simulink model "Model_Main_V2"  (R2019b)
settings: Solver=FixedStepAuto  StartTime=0.0  StopTime=inf  RelTol=1e-3  EnableMultiTasking=on
PreLoadFcn:
  | sampleTime = 0.01;
  | 
  | % Vehicle Parameters
  | R = 0.058;
  | L = 0.1;
  | vehicle = DifferentialDrive(R,L);
  | k = -858.9174;
  | b = 70.9944;
  | %model parameters
  | MODEL_TYPE = 0;
  | MODEL_TYPE_ROAD = 0;
InitFcn:
  | sampleTime = 0.01;
  | 
  | % Vehicle Parameters
  | R = 0.058;
  | L = 0.1;
  | vehicle = DifferentialDrive(R,L);
  | k = -858.9174;
  | b = 70.9944;
undefined symbols (not defined in the file or in its folder): DiscIntNeverNeededParam, InitAngle, InitX
libraries: legoev3lib x5, mobileRoboticsLib x4, aerolibconvert2 x3, simulink x2
settings Model: ExtModeTrigDuration=2  Creator=nikit  LastModifiedBy=nikit
settings SolverCC: PositivePriorityOrder=on
settings OptimizationCC: EnhancedBackFolding=on  PassReuseOutputArgsAs=Individual arguments  ZeroExternalMemoryAtStartup=off  ZeroInternalMemoryAtStartup=off  MaxStackSize=64  OptimizeBlockOrder=speed  DifferentSizesBufferReuse=on  EfficientTunableParamExpr=on
settings DebuggingCC: ParameterTunabilityLossMsg=error
settings HardwareCC: ProdBitPerPointer=32  ProdBitPerSizeT=32  ProdBitPerPtrDiffT=32  ProdLargestAtomicInteger=Long  ProdWordSize=32  ProdHWDeviceType=ARM Compatible->ARM 9
settings SFSimCC: MATLABDynamicMemAlloc=off
settings RTWCC: SystemTargetFile=ert.tlc  HardwareBoard=LEGO MINDSTORMS EV3  TLCOptions="-aInlineSetEventsForThisBaseRateFcn=TLC_FALSE -aSuppressMultiTaskScheduler=TLC_FALSE  -aRateBasedStepFcn=0"  TemplateMakefile=ert_default_tmf  GenerateReport=on  Toolchain=Sourcery G++ Lite v2009q3  IncludeHyperlinkInReport=on  LaunchReport=on  GenerateTraceInfo=on  GenerateTraceReport=on  GenerateTraceReportSl=on  GenerateTraceReportSf=on  GenerateTraceReportEml=on
settings CodeAppCC: ForceParamTrailComments=on  IgnoreCustomStorageClasses=off  OperatorAnnotations=on  SimulinkDataObjDesc=on  SFDataObjDesc=on  InsertBlockDesc=on
settings ERTTargetCC: SupportContinuousTime=on  SupportVariableSizeSignals=on

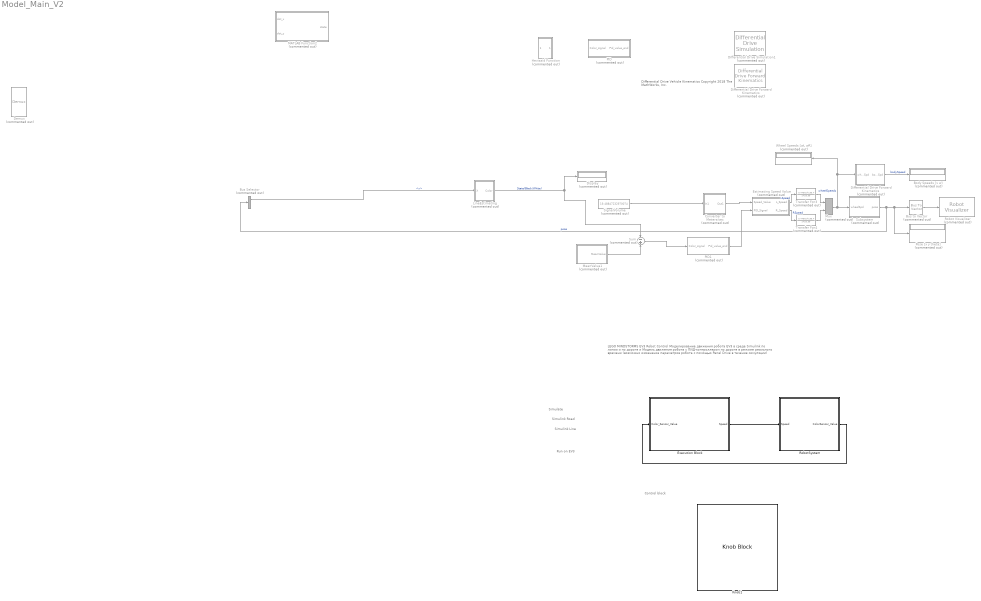
== system Model_Main_V2 ==
  note: LEGO MINDSTORMS EV3 Robot Control
      | Моделирование движения робота EV3 в среде Simulink по линии и по дороге
      | и
      | Модель движения робота с ПИД-контроллером по дороге в режиме реального времени
      | (возможно изменение параметров робота с помощью Panel Drive в течение симуляции)
  note: Simulate
  note: Run on EV3
  note: Simulink Road
  note: Control block
  note: Differential Drive Vehicle Kinematics
      |
      | Copyright 2018 The MathWorks, Inc.
  note: Simulink Line
  Body Speeds [v w] : Display  Commented=on
  Bus Selector : BusSelector  Commented=on  OutputSignals=x,y,ang
  Bus to Vector : BusToVector  Commented=on
  Converter to Meters/sec : Subsystem  Commented=on
  Demux : Demux  Commented=on  Outputs=3
  Differential Drive Forward Kinematics : mobileRoboticsLib/Kinematic Models/Differential Drive/Differential Drive Forward Kinematics  Commented=on  wheelRadius=R  wheelBase=L
      settings: SourceProductName=Mobile Robotics Simulation Library
  Differential Drive Forward Kinematics : Subsystem  Commented=on  AncestorBlock=mobileRoboticsLib/Kinematic Models/Differential Drive/Differential Drive Forward Kinematics  mask(Differential Drive Forward Kinematics){wheelRadius=R, wheelBase=L}
      mask prompts: wheelRadius "Wheel Radius [m]"; wheelBase "Wheelbase [m]"
      mask help:
      | Calculates the forward kinematics for a differential drive vehicle.
      |
      | Input: [wL; wR], the left and right wheel speeds (rad/s)
      |
      | Output: [v; w], the linear (m/s) and angular (rad/s) velocities of the vehicle
      mask Help: web('matlab:edit mrsDocDifferentialDrive')
  Differential Drive Simulation1 : mobileRoboticsLib/Kinematic Models/Differential Drive/Differential Drive Simulation  Commented=on  wheelRadius=R  wheelBase=L  initX=0  initY=18  initAngle=0  Ts=0.01
      link override Differential Drive  Forward Kinematics: wheelRadius=R  wheelBase=L
      link override Generic Robot Simulation: initX=initX  initY=initY  initAngle=initAngle
      settings: SourceProductName=Mobile Robotics Simulation Library
  Display : Display  Commented=on
  Estimating Speed Value : Subsystem  Commented=on
  Execution Block : Subsystem
      mask Display: image('ev3_computer.jpg'); % Use "Edit Image" on toolstrip to change.
  "Hevisaid Function " : Subsystem  Commented=on
  Knob1 : KnobBlock
  LineEstimating : Subsystem  Commented=on
  MATLAB Function2 : MATLAB Function  Commented=on  TreatAsAtomicUnit=on
  MeanValue1 : Subsystem  Commented=on  mask{BlackCode=3, WhiteCode=32}
      mask prompts: BlackCode "BlackColorCode"; WhiteCode "WhiteColorCode"
  Mux : Mux  Commented=on  Inputs=2
  PID : Subsystem  Commented=on
  PID1 : Subsystem  Commented=on
  Pose [x y theta] : Display  Commented=on
  Robot Visualizer : mobileRoboticsLib/Environments/Robot Visualizer  Priority=99  Commented=on  robotRadius=0.15  mapName=map  showTrajectory=on  hasWaypoints=off  hasLidar=off  sensorOffset=[ 0 0 ]  scanAngles=scanAngles  hasObjDetector=off  objDetectorOffset=[ 0, 0 ]  objDetectorAngle=0  objDetectorFOV=pi/4  objDetectorMaxRange=5  objectColors=[ 1, 0, 0; 0, 1, 0; 0, 0, 1 ]  objectMarkers=s
      settings: SourceProductName=Mobile Robotics Simulation Library
  RobotSystem : Subsystem  Variant=on  VariantControl=Variant1
      mask Display:
      | if evalin('base','MODEL_TYPE == 1')
      |     image('EV3_Robot.jpg')
      | else
      |     image('ev3_simulink_sign.jpg')
      | end
  SignalVolume : Constant  Commented=on  Value=19.48847232970074
  Subsystem : Subsystem  Commented=on  mask{R=0.058, L=0.155, InitialX=0.6455, InitialY=0.02, InitialAngle=pi/2, SampleTime=0.01}
      mask prompts: R "WheelR"; L "BodyL"; InitialAngle "InitialAng"; SampleTime "Sample Time"
  Sum : Sum  Commented=on  Inputs=-+
  Transfer Fcn3 : TransferFcn  Commented=on  Numerator=[0.4456 195.4]  Denominator=[1 20.39]
  Transfer Fcn4 : TransferFcn  Commented=on  Numerator=[0.4456 195.4]  Denominator=[1 20.39]
  Wheel Speeds [wL wR] : Display  Commented=on
  wires:
  LineEstimating/1(Color) -> Sum/1, Display/1  "State(Black/White)"
  MeanValue1/1(MeanValue) -> Sum/2
  Estimating Speed Value/1(L_Speed) -> Transfer Fcn3/1  "LSpeed"
  Estimating Speed Value/2(R_Speed) -> Transfer Fcn4/1  "RSpeed"
  Differential Drive Forward Kinematics/1(bodySpd) -> Body Speeds [v w]/1  "bodySpeed"
  Mux/1 -> Subsystem/1(wheelSpd), Differential Drive Forward Kinematics/1(wheelSpd), Wheel Speeds [wL wR]/1  "wheelSpeeds"
  Subsystem/1(pose) -> Pose [x y theta]/1, Bus to Vector/1, Bus Selector/1  "pose"
  Converter to Meters/sec/1(Out1) -> Estimating Speed Value/1(Speed_Value)
  Bus to Vector/1 -> Robot Visualizer/1
  PID1/1(Pid_value_end) -> Estimating Speed Value/2(PID_Signal)
  Bus Selector/1 -> LineEstimating/1(X)  "<x>"
  Sum/1 -> PID1/1(Color_signal)
  SignalVolume/1 -> Converter to Meters/sec/1(In1)
  Transfer Fcn3/1 -> Mux/1
  Transfer Fcn4/1 -> Mux/2
  RobotSystem/1(ColorSensor_Value) -> Execution Block/1(Color_Sensor_Value)
  Execution Block/1(Speed) -> RobotSystem/1(Speed)

== system Model_Main_V2/Converter to Meters//sec ==
  In1 : Inport
  Angle Conversion : aerolibconvert2/Angle Conversion  IU=deg  OU=rad
  Radius : Gain  Gain=R
  Out1 : Outport
  wires:
  Radius/1 -> Out1/1
  Angle Conversion/1 -> Radius/1
  In1/1 -> Angle Conversion/1

== system Model_Main_V2/Differential Drive Forward Kinematics ==
  wheelSpd : Inport
  Demux : Demux  Outputs=2
  ForwardKinematics : Subsystem
  Mux : Mux  Inputs=2
  bodySpd : Outport  VectorParamsAs1DForOutWhenUnconnected=off
  wires:
  Demux/2 -> ForwardKinematics/2(wR)  "wR"
  Demux/1 -> ForwardKinematics/1(wL)  "wL"
  wheelSpd/1 -> Demux/1
  Mux/1 -> bodySpd/1
  ForwardKinematics/2(w) -> Mux/2  "w"
  ForwardKinematics/1(v) -> Mux/1  "v"

== system Model_Main_V2/Estimating Speed Value ==
  note: Estimating Speed Value for each engine taking into account PID_value
  Speed_Value : Inport
  PID_Signal : Inport  Port=2
  Sum1 : Sum  Inputs=+-|
  Sum2 : Sum  Inputs=++|
  L_Speed : Outport
  R_Speed : Outport  Port=2
  wires:
  Speed_Value/1 -> Sum2/1, Sum1/1
  PID_Signal/1 -> Sum2/2, Sum1/2
  Sum2/1 -> R_Speed/1
  Sum1/1 -> L_Speed/1

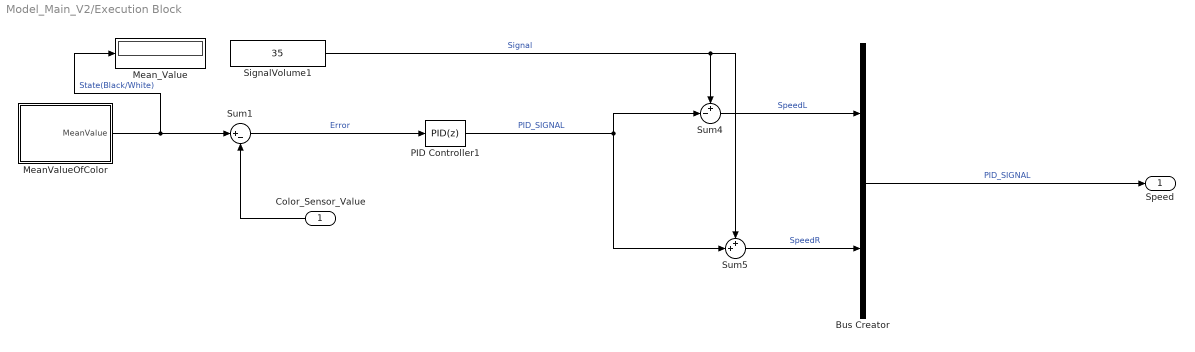
== system Model_Main_V2/Execution Block ==
  Color_Sensor_Value : Inport
  Bus Creator : BusCreator  Inputs=2
  MeanValueOfColor : Subsystem  mask{BlackCode=3, WhiteCode=32}
      mask prompts: BlackCode "BlackColorCode"; WhiteCode "WhiteColorCode"
  Mean_Value : Display
  PID Controller1 : simulink/Continuous/PID Controller  Controller=PID  Form=Parallel  TimeDomain=Discrete-time  SampleTime=0.01  IntegratorMethod=Forward Euler  FilterMethod=Forward Euler  ControllerParametersSource=internal  P=2  I=0.001  D=0.06  UseFilter=off  N=9.96704148788016  TunerSelectOption=Transfer Function Based (PID Tuner App)  InitialConditionSource=internal  InitialConditionForIntegrator=0  InitialConditionForFilter=0  DifferentiatorICPrevScaledInput=0  ExternalReset=none  TrackingMode=off  Kt=1  LimitOutput=off  UpperSaturationLimit=inf  LowerSaturationLimit=-inf  LinearizeAsGain=on  AntiWindupMode=none  Kb=1  POutMin=[]  POutMax=[]  IOutMin=[]  IOutMax=[]  DOutMin=[]  DOutMax=[]  NOutMin=[]  NOutMax=[]  SumOutMin=[]  SumOutMax=[]  SaturationOutMin=[]  SaturationOutMax=[]  PParamMin=[]  PParamMax=[]  IParamMin=[]  IParamMax=[]  DParamMin=[]  DParamMax=[]  NParamMin=[]  NParamMax=[]  KbParamMin=[]  KbParamMax=[]  KtParamMin=[]  KtParamMax=[]  KbOutMin=[]  KbOutMax=[]  KtOutMin=[]  KtOutMax=[]  IntegratorOutMin=[]  IntegratorOutMax=[]  FilterOutMin=[]  FilterOutMax=[]  SumI1OutMin=[]  SumI1OutMax=[]  SumI2OutMin=[]  SumI2OutMax=[]  SumI3OutMin=[]  SumI3OutMax=[]  SumI4OutMin=[]  SumI4OutMax=[]  SumDOutMin=[]  SumDOutMax=[]  DifferentiatorOutMin=[]  DifferentiatorOutMax=[]  FilterDiffOutCoefMin=[]  FilterDiffOutCoefMax=[]  ReciprocalOutMin=[]  ReciprocalOutMax=[]  SumDenOutMin=[]  SumDenOutMax=[]  SumNumOutMin=[]  SumNumOutMax=[]  DivideOutMin=[]  DivideOutMax=[]  IntegratorContinuousStateAttributes=''  IntegratorStateMustResolveToSignalObject=off  IntegratorRTWStateStorageClass=Auto  FilterContinuousStateAttributes=''  FilterStateMustResolveToSignalObject=off  FilterRTWStateStorageClass=Auto  ParallelPVariant=InternalParameters  IdealPVariant=Disabled  IVariant=InternalParameters  DVariant=InternalParameters  IntegratorVariant=Discrete  SatVariant=Disabled  AWVariant=Passthrough  PCopyVariant=Disabled  TRVariant=Disabled  FdbkBlocksVariant=Forward  IdealPFdbkVariant=Disabled  SatFdbkVariant=Disabled  DerivativeFilterVariant=Differentiator  NVariant=Passthrough  NCopyVariant=Disabled_SignalSpec  FilterICVariant=InternalICsDifferentiator  IntegratorICVariant=InternalICs  ExternalResetVariant=Disabled  TRSumVariant=Passthrough  SumFdbkVariant=Disabled  SumVariant=Sum_PID
  SignalVolume1 : Constant  Value=35
  Sum1 : Sum  Inputs=|+-
  Sum4 : Sum  Inputs=+-|
  Sum5 : Sum  Inputs=++|
  Speed : Outport
  wires:
  Sum1/1 -> PID Controller1/1  "Error"
  MeanValueOfColor/1(MeanValue) -> Mean_Value/1, Sum1/1  "State(Black/White)"
  SignalVolume1/1 -> Sum4/1, Sum5/1  "Signal"
  Sum4/1 -> Bus Creator/1  "SpeedL"
  Sum5/1 -> Bus Creator/2  "SpeedR"
  Color_Sensor_Value/1 -> Sum1/2
  Bus Creator/1 -> Speed/1  "PID_SIGNAL"
  PID Controller1/1 -> Sum5/2, Sum4/2  "PID_SIGNAL"

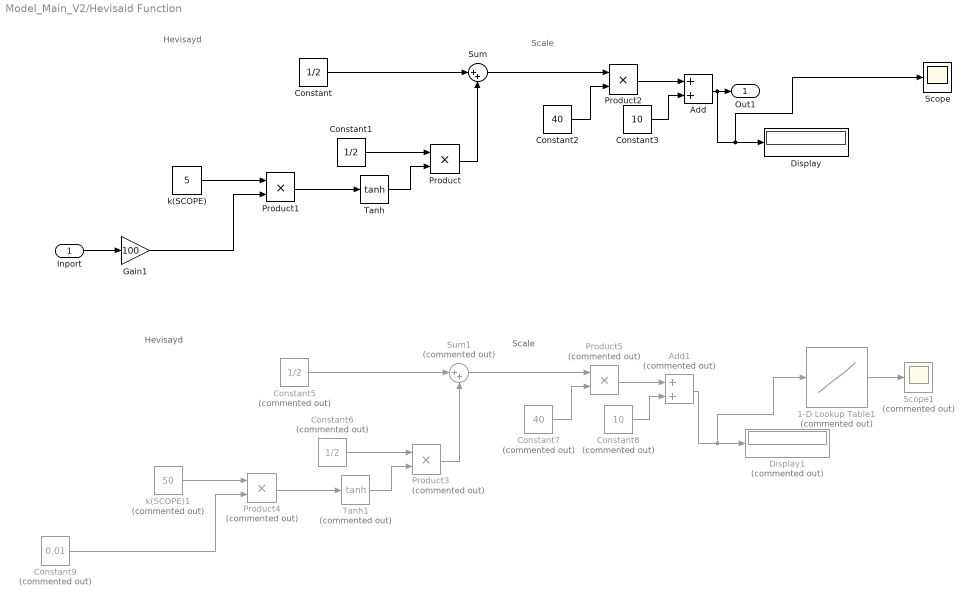
== system Model_Main_V2/Hevisaid Function  ==
  note: Scale
  note: Hevisayd
  note: Scale
  note: Hevisayd
  Inport : Inport
  1-D Lookup Table1 : Lookup_n-D  Commented=on  NumberOfTableDimensions=1  BreakpointsForDimension1=[-5:5]  Table=tanh([-5:5])  InternalRulePriority=Speed  RndMeth=Simplest  InputSameDT=on
  Add : Sum
  Add1 : Sum  Commented=on
  Constant : Constant  Value=1/2
  Constant1 : Constant  Value=1/2
  Constant2 : Constant  Value=40
  Constant3 : Constant  Value=10
  Constant5 : Constant  Commented=on  Value=1/2
  Constant6 : Constant  Commented=on  Value=1/2
  Constant7 : Constant  Commented=on  Value=40
  Constant8 : Constant  Commented=on  Value=10
  Constant9 : Constant  Commented=on  Value=0.01
  Display : Display
  Display1 : Display  Commented=on
  Gain1 : Gain  Gain=100
  Product : Product
  Product1 : Product
  Product2 : Product
  Product3 : Product  Commented=on
  Product4 : Product  Commented=on
  Product5 : Product  Commented=on
  Scope : Scope
  Scope1 : Scope  Commented=on
  Sum : Sum  Inputs=|++
  Sum1 : Sum  Commented=on  Inputs=|++
  Tanh : Trigonometry  Operator=tanh
  Tanh1 : Trigonometry  Commented=on  Operator=tanh
  k(SCOPE) : Constant  Value=5
  k(SCOPE)1 : Constant  Commented=on  Value=50
  Out1 : Outport
  wires:
  Tanh/1 -> Product/2
  Constant/1 -> Sum/1
  Inport/1 -> Gain1/1
  k(SCOPE)/1 -> Product1/1
  Constant2/1 -> Product2/2
  Constant3/1 -> Add/2
  Constant1/1 -> Product/1
  Product/1 -> Sum/2
  Sum/1 -> Product2/1
  Product1/1 -> Tanh/1
  Product2/1 -> Add/1
  Add/1 -> Scope/1, Display/1, Out1/1
  1-D Lookup Table1/1 -> Scope1/1
  Add1/1 -> Display1/1, 1-D Lookup Table1/1
  Product5/1 -> Add1/1
  Product4/1 -> Tanh1/1
  Sum1/1 -> Product5/1
  Product3/1 -> Sum1/2
  Constant6/1 -> Product3/1
  Constant8/1 -> Add1/2
  Constant7/1 -> Product5/2
  k(SCOPE)1/1 -> Product4/1
  Constant9/1 -> Product4/2
  Constant5/1 -> Sum1/1
  Tanh1/1 -> Product3/2
  Gain1/1 -> Product1/2

== system Model_Main_V2/LineEstimating ==
  X : Inport
  Add : Sum
  Constant : Constant  Value=k
  Constant1 : Constant  Value=b
  Product : Product
  Saturation : Saturate  UpperLimit=32  LowerLimit=3
  Color : Outport
  wires:
  Constant1/1 -> Add/2
  Constant/1 -> Product/2
  Add/1 -> Saturation/1
  Product/1 -> Add/1
  X/1 -> Product/1
  Saturation/1 -> Color/1

== system Model_Main_V2/MeanValue1 ==
  Subsystem : Subsystem  mask(Find mean value of two colors){Black=BlackCode, White=WhiteCode}
      mask prompts: Black "BlackColorCode"; White "WhiteColorCode"
      mask help: You need to write codes of two colors to find mean value
  MeanValue : Outport
  wires:
  Subsystem/1(MeanValue) -> MeanValue/1

== system Model_Main_V2/PID ==
  Color_signal : Inport
  Der_koef : Gain  Gain=0
  Derivative : Derivative
  Integral : Gain  Gain=5.999999999999999e-08
  Integrator : Integrator
  Proportional : Gain  Gain=0.6
  Sum : Sum  Inputs=+++
  Pid_value_end : Outport
  wires:
  Sum/1 -> Pid_value_end/1
  Color_signal/1 -> Integral/1, Der_koef/1, Proportional/1
  Integrator/1 -> Sum/2
  Derivative/1 -> Sum/3
  Der_koef/1 -> Derivative/1
  Proportional/1 -> Sum/1
  Integral/1 -> Integrator/1

== system Model_Main_V2/PID1 ==
  Color_signal : Inport
  PID Controller : simulink/Continuous/PID Controller  Controller=PID  Form=Parallel  TimeDomain=Continuous-time  SampleTime=-1  IntegratorMethod=Forward Euler  FilterMethod=Forward Euler  ControllerParametersSource=internal  P=0.106625032301166  I=0.00220549691350034  D=0  UseFilter=on  N=405.197736313364  TunerSelectOption=Transfer Function Based (PID Tuner App)  InitialConditionSource=internal  InitialConditionForIntegrator=0  InitialConditionForFilter=0  DifferentiatorICPrevScaledInput=0  ExternalReset=none  TrackingMode=off  Kt=1  LimitOutput=off  UpperSaturationLimit=inf  LowerSaturationLimit=-inf  LinearizeAsGain=on  AntiWindupMode=none  Kb=1  POutMin=[]  POutMax=[]  IOutMin=[]  IOutMax=[]  DOutMin=[]  DOutMax=[]  NOutMin=[]  NOutMax=[]  SumOutMin=[]  SumOutMax=[]  SaturationOutMin=[]  SaturationOutMax=[]  PParamMin=[]  PParamMax=[]  IParamMin=[]  IParamMax=[]  DParamMin=[]  DParamMax=[]  NParamMin=[]  NParamMax=[]  KbParamMin=[]  KbParamMax=[]  KtParamMin=[]  KtParamMax=[]  KbOutMin=[]  KbOutMax=[]  KtOutMin=[]  KtOutMax=[]  IntegratorOutMin=[]  IntegratorOutMax=[]  FilterOutMin=[]  FilterOutMax=[]  SumI1OutMin=[]  SumI1OutMax=[]  SumI2OutMin=[]  SumI2OutMax=[]  SumI3OutMin=[]  SumI3OutMax=[]  SumI4OutMin=[]  SumI4OutMax=[]  SumDOutMin=[]  SumDOutMax=[]  DifferentiatorOutMin=[]  DifferentiatorOutMax=[]  FilterDiffOutCoefMin=[]  FilterDiffOutCoefMax=[]  ReciprocalOutMin=[]  ReciprocalOutMax=[]  SumDenOutMin=[]  SumDenOutMax=[]  SumNumOutMin=[]  SumNumOutMax=[]  DivideOutMin=[]  DivideOutMax=[]  IntegratorContinuousStateAttributes=''  IntegratorStateMustResolveToSignalObject=off  IntegratorRTWStateStorageClass=Auto  FilterContinuousStateAttributes=''  FilterStateMustResolveToSignalObject=off  FilterRTWStateStorageClass=Auto  ParallelPVariant=InternalParameters  IdealPVariant=Disabled  IVariant=InternalParameters  DVariant=InternalParameters  IntegratorVariant=Continuous  SatVariant=Disabled  AWVariant=Passthrough  PCopyVariant=Disabled  TRVariant=Disabled  FdbkBlocksVariant=Forward  IdealPFdbkVariant=Disabled  SatFdbkVariant=Disabled  DerivativeFilterVariant=ContFilter  NVariant=InternalParameters  NCopyVariant=Disabled  FilterICVariant=InternalICsFilter  IntegratorICVariant=InternalICs  ExternalResetVariant=Disabled  TRSumVariant=Passthrough  SumFdbkVariant=Disabled  SumVariant=Sum_PID
  Pid_value_end : Outport
  wires:
  Color_signal/1 -> PID Controller/1
  PID Controller/1 -> Pid_value_end/1

== system Model_Main_V2/RobotSystem ==
  Speed : Inport
  RealModel : Subsystem  VariantControl=MODEL_TYPE == 1
      mask Display: image('EV3_Robot.jpg'); % Use "Edit Image" on toolstrip to change.
  SimulinkModel : Subsystem  VariantControl=(default)
      mask Display: image('ev3_simulink_sign.jpg'); % Use "Edit Image" on toolstrip to change.
  ColorSensor_Value : Outport

== system Model_Main_V2/Subsystem ==
  wheelSpd : Inport
  Differential Drive Forward Kinematics : Subsystem  AncestorBlock=mobileRoboticsLib/Kinematic Models/Differential Drive/Differential Drive Forward Kinematics  mask(Differential Drive Forward Kinematics){wheelRadius=R, wheelBase=L}
      mask prompts: wheelRadius "Wheel Radius [m]"; wheelBase "Wheelbase [m]"
      mask help:
      | Calculates the forward kinematics for a differential drive vehicle.
      |
      | Input: [wL; wR], the left and right wheel speeds (rad/s)
      |
      | Output: [v; w], the linear (m/s) and angular (rad/s) velocities of the vehicle
      mask Help: web('matlab:edit mrsDocDifferentialDrive')
  Generoc Robot Simulator : Subsystem  mask{initX=InitialX, initY=InitialY, initAngle=InitialAngle, Ts=SampleTime}
      mask prompts: initX "InitialX"; initY "InitialY"; initAngle "InitialAngle"; Ts "SampleTime"
  Subsystem : Subsystem
  pose : Outport
  wires:
  Generoc Robot Simulator/1(pose) -> pose/1
  wheelSpd/1 -> Differential Drive Forward Kinematics/1(wheelSpd)
  Differential Drive Forward Kinematics/1(bodySpd) -> Subsystem/1(In1)
  Subsystem/1(Out1) -> Generoc Robot Simulator/1(Speed)

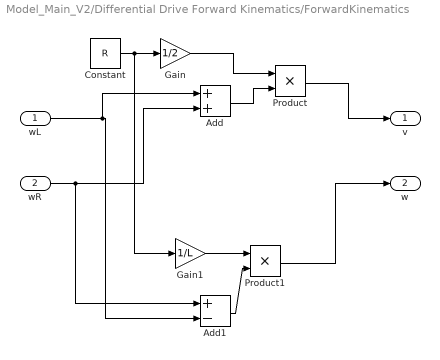
== system Model_Main_V2/Differential Drive Forward Kinematics/ForwardKinematics ==
  wL : Inport
  wR : Inport  Port=2
  Add : Sum
  Add1 : Sum  Inputs=+-
  Constant : Constant  Value=R
  Gain : Gain  Gain=1/2
  Gain1 : Gain  Gain=1/L
  Product : Product
  Product1 : Product
  v : Outport
  w : Outport  Port=2
  wires:
  wL/1 -> Add1/2, Add/1
  Product/1 -> v/1
  Constant/1 -> Gain1/1, Gain/1
  wR/1 -> Add1/1, Add/2
  Add/1 -> Product/2
  Product1/1 -> w/1
  Gain1/1 -> Product1/1
  Gain/1 -> Product/1
  Add1/1 -> Product1/2

== system Model_Main_V2/Execution Block/MeanValueOfColor ==
  Subsystem : Subsystem  mask(Find mean value of two colors){Black=BlackCode, White=WhiteCode}
      mask prompts: Black "BlackColorCode"; White "WhiteColorCode"
      mask help: You need to write codes of two colors to find mean value
  MeanValue : Outport
  wires:
  Subsystem/1(MeanValue) -> MeanValue/1

== system Model_Main_V2/MeanValue1/Subsystem ==
  Add : Sum  OutDataTypeStr=int8
  Black : Constant  Value=White
  Constant : Constant  Value=2
  Divide : Product  Inputs=*/
  White : Constant  Value=Black
  MeanValue : Outport
  wires:
  Black/1 -> Add/1
  Divide/1 -> MeanValue/1
  White/1 -> Add/2
  Constant/1 -> Divide/2
  Add/1 -> Divide/1

== system Model_Main_V2/RobotSystem/RealModel ==
  Speed : Inport
  Bus Selector : BusSelector  OutputSignals=SpeedL,SpeedR
  ColorSensor : Subsystem
      mask Display: image('ev3_color_sensor.png'); % Use "Edit Image" on toolstrip to change.
  Display_L : legoev3lib/Display  slcdStr=Left  slcdLine=1  slcdFormat=Decimal
      settings: SourceProductName=Simulink Support Package for LEGO MINDSTORMS EV3 Hardware  SourceProductBaseCode=LEGOEV3
  Display_R : legoev3lib/Display  slcdStr=Right  slcdLine=2  slcdFormat=Decimal
      settings: SourceProductName=Simulink Support Package for LEGO MINDSTORMS EV3 Hardware  SourceProductBaseCode=LEGOEV3
  Left1 : legoev3lib/Motor  sportNumber=A  sstopAction=Brake
  Right1 : legoev3lib/Motor  sportNumber=D  sstopAction=Brake
  WheelSpeedsScope : Scope  Commented=on  NumInputPorts=2
  ColorSensor_Value : Outport
  wires:
  Bus Selector/1 -> WheelSpeedsScope/1, Display_L/1, Left1/1  "<SpeedL>"
  Speed/1 -> Bus Selector/1
  Bus Selector/2 -> Display_R/1, WheelSpeedsScope/2, Right1/1  "<SpeedR>"
  ColorSensor/1("Color ") -> ColorSensor_Value/1

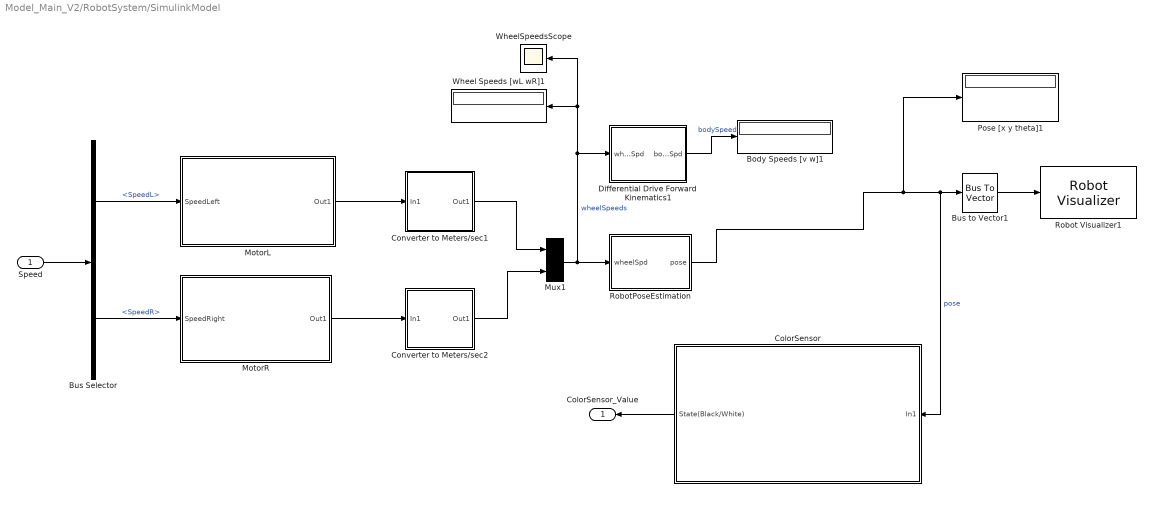
== system Model_Main_V2/RobotSystem/SimulinkModel ==
  Speed : Inport
  Body Speeds [v w]1 : Display
  Bus Selector : BusSelector  OutputSignals=SpeedL,SpeedR
  Bus to Vector1 : BusToVector
  ColorSensor : Subsystem
      mask Display: image('ev3_color_sensor.png'); % Use "Edit Image" on toolstrip to change.
  Converter to Meters/sec1 : Subsystem
      mask Display: image('ev3_converter_sign.png'); % Use "Edit Image" on toolstrip to change.
  Converter to Meters/sec2 : Subsystem
      mask Display: image('ev3_converter_sign.png'); % Use "Edit Image" on toolstrip to change.
  Differential Drive Forward Kinematics1 : Subsystem  AncestorBlock=mobileRoboticsLib/Kinematic Models/Differential Drive/Differential Drive Forward Kinematics  mask(Differential Drive Forward Kinematics){wheelRadius=R, wheelBase=L}
      mask prompts: wheelRadius "Wheel Radius [m]"; wheelBase "Wheelbase [m]"
      mask help:
      | Calculates the forward kinematics for a differential drive vehicle.
      |
      | Input: [wL; wR], the left and right wheel speeds (rad/s)
      |
      | Output: [v; w], the linear (m/s) and angular (rad/s) velocities of the vehicle
      mask Help: web('matlab:edit mrsDocDifferentialDrive')
  MotorL : Subsystem
      mask Display: image('ev3_motor.jpg'); % Use "Edit Image" on toolstrip to change.
  MotorR : Subsystem
      mask Display: image('ev3_motor.jpg'); % Use "Edit Image" on toolstrip to change.
  Mux1 : Mux  Inputs=2
  Pose [x y theta]1 : Display
  Robot Visualizer1 : mobileRoboticsLib/Environments/Robot Visualizer  Priority=99  robotRadius=0.15  mapName=map  showTrajectory=on  hasWaypoints=off  hasLidar=off  sensorOffset=[ 0 0 ]  scanAngles=scanAngles  hasObjDetector=off  objDetectorOffset=[ 0, 0 ]  objDetectorAngle=0  objDetectorFOV=pi/4  objDetectorMaxRange=5  objectColors=[ 1, 0, 0; 0, 1, 0; 0, 0, 1 ]  objectMarkers=s
      settings: SourceProductName=Mobile Robotics Simulation Library
  RobotPoseEstimation : Subsystem  mask{R=0.058, L=0.155, InitialX=InitX, InitialY=0.02, InitialAngle=InitAngle, SampleTime=0.01}
      mask prompts: R "WheelR"; L "BodyL"; InitialAngle "InitialAng"; SampleTime "Sample Time"
  Wheel Speeds [wL wR]1 : Display
  WheelSpeedsScope : Scope
  ColorSensor_Value : Outport
  wires:
  Mux1/1 -> RobotPoseEstimation/1(wheelSpd), WheelSpeedsScope/1, Wheel Speeds [wL wR]1/1, Differential Drive Forward Kinematics1/1(wheelSpd)  "wheelSpeeds"
  Differential Drive Forward Kinematics1/1(bodySpd) -> Body Speeds [v w]1/1  "bodySpeed"
  Converter to Meters/sec1/1(Out1) -> Mux1/1
  Converter to Meters/sec2/1(Out1) -> Mux1/2
  RobotPoseEstimation/1(pose) -> Pose [x y theta]1/1, ColorSensor/1(In1), Bus to Vector1/1  "pose"
  Bus to Vector1/1 -> Robot Visualizer1/1
  MotorL/1(Out1) -> Converter to Meters/sec1/1(In1)
  MotorR/1(Out1) -> Converter to Meters/sec2/1(In1)
  Speed/1 -> Bus Selector/1
  Bus Selector/1 -> MotorL/1(SpeedLeft)  "<SpeedL>"
  Bus Selector/2 -> MotorR/1(SpeedRight)  "<SpeedR>"
  ColorSensor/1(State(Black/White)) -> ColorSensor_Value/1

== system Model_Main_V2/Subsystem/Differential Drive Forward Kinematics ==
  wheelSpd : Inport
  Bus Creator : BusCreator  Inputs=2
  Demux : Demux  Outputs=2
  ForwardKinematics : Subsystem
  bodySpd : Outport  VectorParamsAs1DForOutWhenUnconnected=off
  wires:
  Demux/2 -> ForwardKinematics/2(wR)  "wR"
  Demux/1 -> ForwardKinematics/1(wL)  "wL"
  wheelSpd/1 -> Demux/1
  Bus Creator/1 -> bodySpd/1
  ForwardKinematics/2(w) -> Bus Creator/2  "w"
  ForwardKinematics/1(v) -> Bus Creator/1  "v"

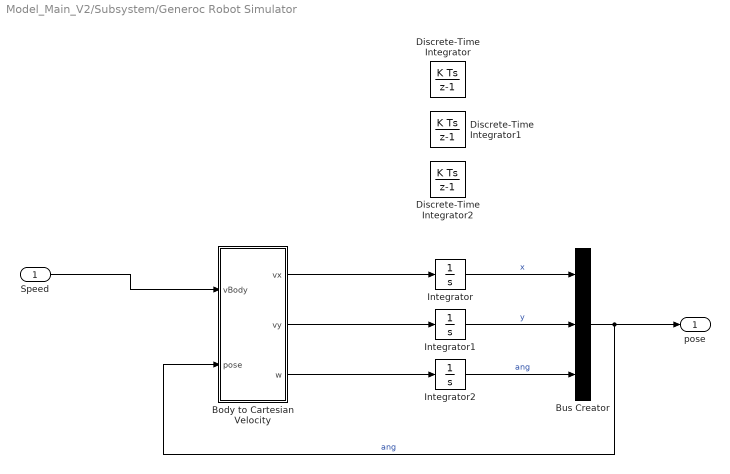
== system Model_Main_V2/Subsystem/Generoc Robot Simulator ==
  Speed : Inport
  Body to Cartesian Velocity : Subsystem  mask(Body to World Velocity){}
      mask help:
      | Converts a 2D velocity input [vx;vy;w] from body (vehicle) coordinates to world (global) coordinates.
      |
      | vx = Linear velocity in x-direction (longitudinal)
      | vy = Linear velocity in y-direction (lateral)
      | w = Angular velocity (about z-axis)
  Bus Creator : BusCreator  Inputs=3
  Discrete-Time Integrator : DiscreteIntegrator  InitialCondition=initX  SampleTime=Ts  ICPrevOutput=DiscIntNeverNeededParam  ICPrevScaledInput=DiscIntNeverNeededParam
  Discrete-Time Integrator1 : DiscreteIntegrator  InitialCondition=initY  SampleTime=Ts  ICPrevOutput=DiscIntNeverNeededParam  ICPrevScaledInput=DiscIntNeverNeededParam
  Discrete-Time Integrator2 : DiscreteIntegrator  InitialCondition=initAngle  SampleTime=Ts  ICPrevOutput=DiscIntNeverNeededParam  ICPrevScaledInput=DiscIntNeverNeededParam
  Integrator : Integrator  InitialCondition=initX
  Integrator1 : Integrator  InitialCondition=initY
  Integrator2 : Integrator  InitialCondition=InitialAngle
  pose : Outport
  wires:
  Speed/1 -> Body to Cartesian Velocity/1(vBody)
  Body to Cartesian Velocity/3(w) -> Integrator2/1
  Integrator/1 -> Bus Creator/1  "x"
  Integrator1/1 -> Bus Creator/2  "y"
  Body to Cartesian Velocity/1(vx) -> Integrator/1
  Integrator2/1 -> Bus Creator/3  "ang"
  Body to Cartesian Velocity/2(vy) -> Integrator1/1
  Bus Creator/1 -> pose/1, Body to Cartesian Velocity/2(pose)  "ang"

== system Model_Main_V2/Subsystem/Subsystem ==
  In1 : Inport
  Bus Creator : BusCreator  Inputs=3
  Bus Selector : BusSelector  OutputSignals=v,w
  Constant : Constant  Value=0
  Gain : Gain
  Out1 : Outport
  wires:
  Constant/1 -> Bus Creator/2  "vy"
  Bus Selector/1 -> Gain/1  "<v>"
  Bus Creator/1 -> Out1/1
  Bus Selector/2 -> Bus Creator/3  "<w>"
  In1/1 -> Bus Selector/1
  Gain/1 -> Bus Creator/1  "vx"

== system Model_Main_V2/Execution Block/MeanValueOfColor/Subsystem ==
  Add : Sum  OutDataTypeStr=int8
  Black : Constant  Value=White
  Constant : Constant  Value=2
  Divide : Product  Inputs=*/
  White : Constant  Value=Black
  MeanValue : Outport
  wires:
  Add/1 -> Divide/1
  Constant/1 -> Divide/2
  White/1 -> Add/2
  Divide/1 -> MeanValue/1
  Black/1 -> Add/1

== system Model_Main_V2/RobotSystem/RealModel/ColorSensor ==
  Color Sensor : legoev3lib/Color Sensor  portNumber=2  mode=Reflected light intensity  sampleTime=0.01
      settings: SourceProductName=Simulink Support Package for LEGO MINDSTORMS EV3 Hardware  SourceProductBaseCode=LEGOEV3
  Data Type Conversion : DataTypeConversion  OutDataTypeStr=int8
  "Color " : Outport
  wires:
  Data Type Conversion/1 -> "Color "/1  "Color"
  Color Sensor/1 -> Data Type Conversion/1

== system Model_Main_V2/RobotSystem/SimulinkModel/ColorSensor ==
  In1 : Inport
  ColorScope : Scope
  Color_Value : Display
  RegionTracker : Subsystem  Variant=on  VariantControl=Variant1
  State(Black/White) : Outport
  wires:
  RegionTracker/1(Outport) -> ColorScope/1, Color_Value/1, State(Black/White)/1
  In1/1 -> RegionTracker/1(In1)

== system Model_Main_V2/RobotSystem/SimulinkModel/Converter to Meters//sec1 ==
  In1 : Inport
  Angle Conversion : aerolibconvert2/Angle Conversion  IU=deg  OU=rad
  Radius : Gain  Gain=R
  Out1 : Outport
  wires:
  Radius/1 -> Out1/1
  Angle Conversion/1 -> Radius/1
  In1/1 -> Angle Conversion/1

== system Model_Main_V2/RobotSystem/SimulinkModel/Converter to Meters//sec2 ==
  In1 : Inport
  Angle Conversion : aerolibconvert2/Angle Conversion  IU=deg  OU=rad
  Radius : Gain  Gain=R
  Out1 : Outport
  wires:
  In1/1 -> Angle Conversion/1
  Angle Conversion/1 -> Radius/1
  Radius/1 -> Out1/1

== system Model_Main_V2/RobotSystem/SimulinkModel/Differential Drive Forward Kinematics1 ==
  wheelSpd : Inport
  Demux : Demux  Outputs=2
  ForwardKinematics : Subsystem
  Mux : Mux  Inputs=2
  bodySpd : Outport  VectorParamsAs1DForOutWhenUnconnected=off
  wires:
  Demux/2 -> ForwardKinematics/2(wR)  "wR"
  Demux/1 -> ForwardKinematics/1(wL)  "wL"
  wheelSpd/1 -> Demux/1
  Mux/1 -> bodySpd/1
  ForwardKinematics/2(w) -> Mux/2  "w"
  ForwardKinematics/1(v) -> Mux/1  "v"

== system Model_Main_V2/RobotSystem/SimulinkModel/MotorL ==
  SpeedLeft : Inport
  Transfer Fcn2 : TransferFcn  Numerator=[0.4456 195.4]  Denominator=[1 20.39]
  Out1 : Outport
  wires:
  SpeedLeft/1 -> Transfer Fcn2/1
  Transfer Fcn2/1 -> Out1/1

== system Model_Main_V2/RobotSystem/SimulinkModel/MotorR ==
  SpeedRight : Inport
  Transfer Fcn1 : TransferFcn  Numerator=[0.4456 195.4]  Denominator=[1 20.39]
  Out1 : Outport
  wires:
  Transfer Fcn1/1 -> Out1/1
  SpeedRight/1 -> Transfer Fcn1/1

== system Model_Main_V2/RobotSystem/SimulinkModel/RobotPoseEstimation ==
  wheelSpd : Inport
  Differential Drive Forward Kinematics : Subsystem  AncestorBlock=mobileRoboticsLib/Kinematic Models/Differential Drive/Differential Drive Forward Kinematics  mask(Differential Drive Forward Kinematics){wheelRadius=R, wheelBase=L}
      mask prompts: wheelRadius "Wheel Radius [m]"; wheelBase "Wheelbase [m]"
      mask help:
      | Calculates the forward kinematics for a differential drive vehicle.
      |
      | Input: [wL; wR], the left and right wheel speeds (rad/s)
      |
      | Output: [v; w], the linear (m/s) and angular (rad/s) velocities of the vehicle
      mask Help: web('matlab:edit mrsDocDifferentialDrive')
  Generoc Robot Simulator : Subsystem  mask{initX=InitialX, initY=InitialY, initAngle=InitialAngle, Ts=SampleTime}
      mask prompts: initX "InitialX"; initY "InitialY"; initAngle "InitialAngle"; Ts "SampleTime"
  Subsystem : Subsystem
  pose : Outport
  wires:
  Generoc Robot Simulator/1(pose) -> pose/1
  wheelSpd/1 -> Differential Drive Forward Kinematics/1(wheelSpd)
  Differential Drive Forward Kinematics/1(bodySpd) -> Subsystem/1(In1)
  Subsystem/1(Out1) -> Generoc Robot Simulator/1(Speed)

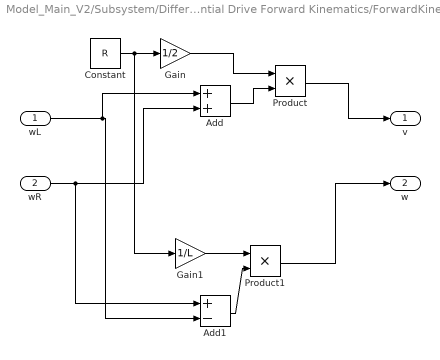
== system Model_Main_V2/Subsystem/Differential Drive Forward Kinematics/ForwardKinematics ==
  wL : Inport
  wR : Inport  Port=2
  Add : Sum
  Add1 : Sum  Inputs=+-
  Constant : Constant  Value=R
  Gain : Gain  Gain=1/2
  Gain1 : Gain  Gain=1/L
  Product : Product
  Product1 : Product
  v : Outport
  w : Outport  Port=2
  wires:
  wL/1 -> Add1/2, Add/1
  Product/1 -> v/1
  Constant/1 -> Gain1/1, Gain/1
  wR/1 -> Add1/1, Add/2
  Add/1 -> Product/2
  Product1/1 -> w/1
  Gain1/1 -> Product1/1
  Gain/1 -> Product/1
  Add1/1 -> Product1/2

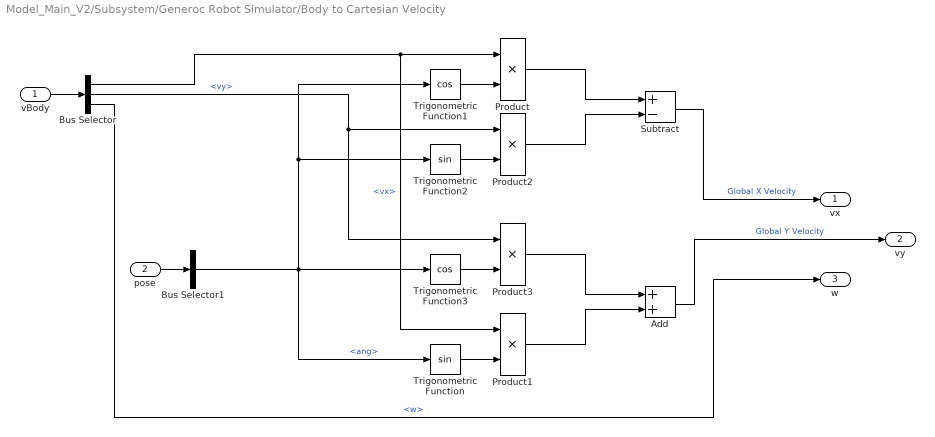
== system Model_Main_V2/Subsystem/Generoc Robot Simulator/Body to Cartesian Velocity ==
  vBody : Inport
  pose : Inport  Port=2
  Add : Sum
  Bus Selector : BusSelector  OutputSignals=vx,vy,w
  Bus Selector1 : BusSelector  OutputSignals=ang
  Product{,1..3} (4 alike) : Product
  Subtract : Sum  Inputs=+-
  Trigonometric Function : Trigonometry
  Trigonometric Function1 : Trigonometry  Operator=cos
  Trigonometric Function2 : Trigonometry
  Trigonometric Function3 : Trigonometry  Operator=cos
  vx : Outport  VectorParamsAs1DForOutWhenUnconnected=off
  vy : Outport  Port=2  VectorParamsAs1DForOutWhenUnconnected=off
  w : Outport  Port=3  VectorParamsAs1DForOutWhenUnconnected=off
  wires:
  Bus Selector/3 -> w/1  "<w>"
  vBody/1 -> Bus Selector/1
  Trigonometric Function/1 -> Product1/2
  Product1/1 -> Add/2
  Product/1 -> Subtract/1
  Trigonometric Function1/1 -> Product/2
  Bus Selector/1 -> Product1/1, Product/1  "<vx>"
  Bus Selector1/1 -> Trigonometric Function3/1, Trigonometric Function2/1, Trigonometric Function1/1, Trigonometric Function/1  "<ang>"
  Subtract/1 -> vx/1  "Global X Velocity"
  Trigonometric Function2/1 -> Product2/2
  Bus Selector/2 -> Product3/1, Product2/1  "<vy>"
  Product2/1 -> Subtract/2
  Trigonometric Function3/1 -> Product3/2
  Product3/1 -> Add/1
  Add/1 -> vy/1  "Global Y Velocity"
  pose/1 -> Bus Selector1/1

== system Model_Main_V2/RobotSystem/SimulinkModel/ColorSensor/RegionTracker ==
  In1 : Inport
  LineSubsystem : Subsystem  VariantControl=(default)
  RegionTracker : Subsystem  VariantControl=MODEL_TYPE_ROAD == 1
  Outport : Outport

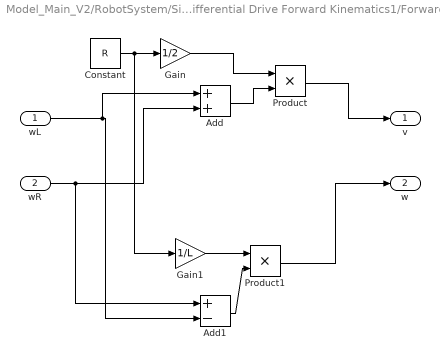
== system Model_Main_V2/RobotSystem/SimulinkModel/Differential Drive Forward Kinematics1/ForwardKinematics ==
  wL : Inport
  wR : Inport  Port=2
  Add : Sum
  Add1 : Sum  Inputs=+-
  Constant : Constant  Value=R
  Gain : Gain  Gain=1/2
  Gain1 : Gain  Gain=1/L
  Product : Product
  Product1 : Product
  v : Outport
  w : Outport  Port=2
  wires:
  wL/1 -> Add1/2, Add/1
  Product/1 -> v/1
  Constant/1 -> Gain1/1, Gain/1
  wR/1 -> Add1/1, Add/2
  Add/1 -> Product/2
  Product1/1 -> w/1
  Gain1/1 -> Product1/1
  Gain/1 -> Product/1
  Add1/1 -> Product1/2

== system Model_Main_V2/RobotSystem/SimulinkModel/RobotPoseEstimation/Differential Drive Forward Kinematics ==
  wheelSpd : Inport
  Bus Creator : BusCreator  Inputs=2
  Demux : Demux  Outputs=2
  ForwardKinematics : Subsystem
  bodySpd : Outport  VectorParamsAs1DForOutWhenUnconnected=off
  wires:
  Demux/2 -> ForwardKinematics/2(wR)  "wR"
  Demux/1 -> ForwardKinematics/1(wL)  "wL"
  wheelSpd/1 -> Demux/1
  Bus Creator/1 -> bodySpd/1
  ForwardKinematics/2(w) -> Bus Creator/2  "w"
  ForwardKinematics/1(v) -> Bus Creator/1  "v"

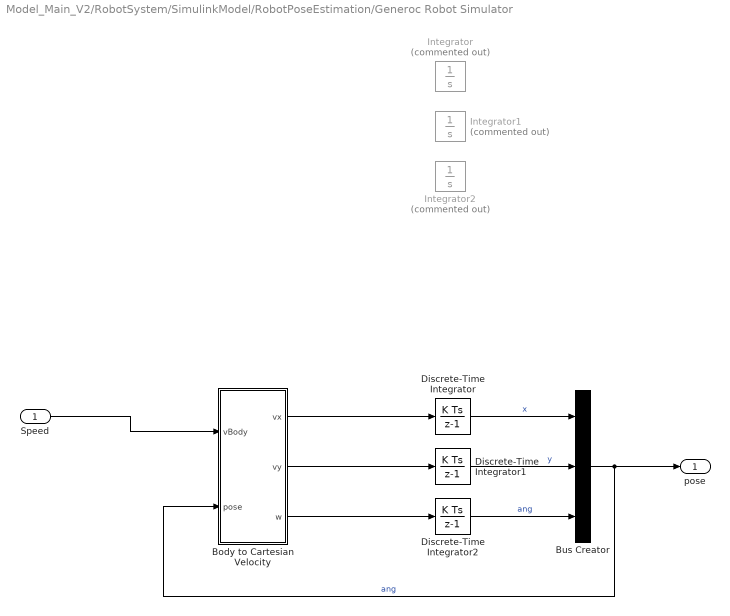
== system Model_Main_V2/RobotSystem/SimulinkModel/RobotPoseEstimation/Generoc Robot Simulator ==
  Speed : Inport
  Body to Cartesian Velocity : Subsystem  mask(Body to World Velocity){}
      mask help:
      | Converts a 2D velocity input [vx;vy;w] from body (vehicle) coordinates to world (global) coordinates.
      |
      | vx = Linear velocity in x-direction (longitudinal)
      | vy = Linear velocity in y-direction (lateral)
      | w = Angular velocity (about z-axis)
  Bus Creator : BusCreator  Inputs=3
  Discrete-Time Integrator : DiscreteIntegrator  InitialCondition=initX  SampleTime=Ts  ICPrevOutput=DiscIntNeverNeededParam  ICPrevScaledInput=DiscIntNeverNeededParam
  Discrete-Time Integrator1 : DiscreteIntegrator  InitialCondition=initY  SampleTime=Ts  ICPrevOutput=DiscIntNeverNeededParam  ICPrevScaledInput=DiscIntNeverNeededParam
  Discrete-Time Integrator2 : DiscreteIntegrator  InitialCondition=initAngle  SampleTime=Ts  ICPrevOutput=DiscIntNeverNeededParam  ICPrevScaledInput=DiscIntNeverNeededParam
  Integrator : Integrator  Commented=on  InitialCondition=initX
  Integrator1 : Integrator  Commented=on  InitialCondition=initY
  Integrator2 : Integrator  Commented=on  InitialCondition=InitialAngle
  pose : Outport
  wires:
  Speed/1 -> Body to Cartesian Velocity/1(vBody)
  Body to Cartesian Velocity/3(w) -> Discrete-Time Integrator2/1
  Discrete-Time Integrator/1 -> Bus Creator/1  "x"
  Discrete-Time Integrator1/1 -> Bus Creator/2  "y"
  Body to Cartesian Velocity/1(vx) -> Discrete-Time Integrator/1
  Discrete-Time Integrator2/1 -> Bus Creator/3  "ang"
  Body to Cartesian Velocity/2(vy) -> Discrete-Time Integrator1/1
  Bus Creator/1 -> pose/1, Body to Cartesian Velocity/2(pose)  "ang"

== system Model_Main_V2/RobotSystem/SimulinkModel/RobotPoseEstimation/Subsystem ==
  In1 : Inport
  Bus Creator : BusCreator  Inputs=3
  Bus Selector : BusSelector  OutputSignals=v,w
  Constant : Constant  Value=0
  Gain : Gain
  Out1 : Outport
  wires:
  Constant/1 -> Bus Creator/2  "vy"
  Bus Selector/1 -> Gain/1  "<v>"
  Bus Creator/1 -> Out1/1
  Bus Selector/2 -> Bus Creator/3  "<w>"
  In1/1 -> Bus Selector/1
  Gain/1 -> Bus Creator/1  "vx"

== system Model_Main_V2/RobotSystem/SimulinkModel/ColorSensor/RegionTracker/LineSubsystem ==
  In1 : Inport
  Bus Selector1 : BusSelector  OutputSignals=x,y,ang
  LineEstimating1 : Subsystem
  Terminator : Terminator
  Terminator1 : Terminator
  Outport : Outport
  wires:
  In1/1 -> Bus Selector1/1
  Bus Selector1/1 -> LineEstimating1/1(X)  "<x>"
  LineEstimating1/1(Color) -> Outport/1  "State(Black/White)"
  Bus Selector1/3 -> Terminator1/1  "<ang>"
  Bus Selector1/2 -> Terminator/1  "<y>"

== system Model_Main_V2/RobotSystem/SimulinkModel/ColorSensor/RegionTracker/RegionTracker ==
  In1 : Inport
  Bus Selector2 : BusSelector  OutputSignals=x,y,ang
  Data Type Conversion : DataTypeConversion  OutDataTypeStr=double
  MATLAB Function : MATLAB Function  TreatAsAtomicUnit=on
  Terminator2 : Terminator
  Outport : Outport
  wires:
  Bus Selector2/3 -> Terminator2/1  "<ang>"
  In1/1 -> Bus Selector2/1
  Bus Selector2/2 -> MATLAB Function/2(dot_y)  "<y>"
  Bus Selector2/1 -> MATLAB Function/1(dot_x)  "<x>"
  MATLAB Function/1(stateC) -> Data Type Conversion/1  "State(Black/White)"
  Data Type Conversion/1 -> Outport/1

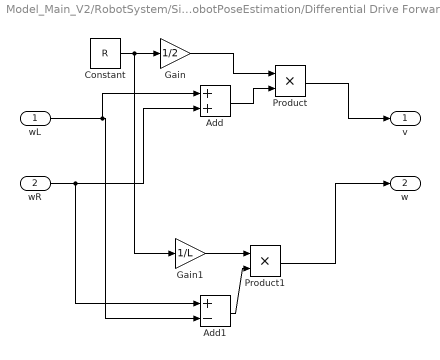
== system Model_Main_V2/RobotSystem/SimulinkModel/RobotPoseEstimation/Differential Drive Forward Kinematics/ForwardKinematics ==
  wL : Inport
  wR : Inport  Port=2
  Add : Sum
  Add1 : Sum  Inputs=+-
  Constant : Constant  Value=R
  Gain : Gain  Gain=1/2
  Gain1 : Gain  Gain=1/L
  Product : Product
  Product1 : Product
  v : Outport
  w : Outport  Port=2
  wires:
  wL/1 -> Add1/2, Add/1
  Product/1 -> v/1
  Constant/1 -> Gain1/1, Gain/1
  wR/1 -> Add1/1, Add/2
  Add/1 -> Product/2
  Product1/1 -> w/1
  Gain1/1 -> Product1/1
  Gain/1 -> Product/1
  Add1/1 -> Product1/2

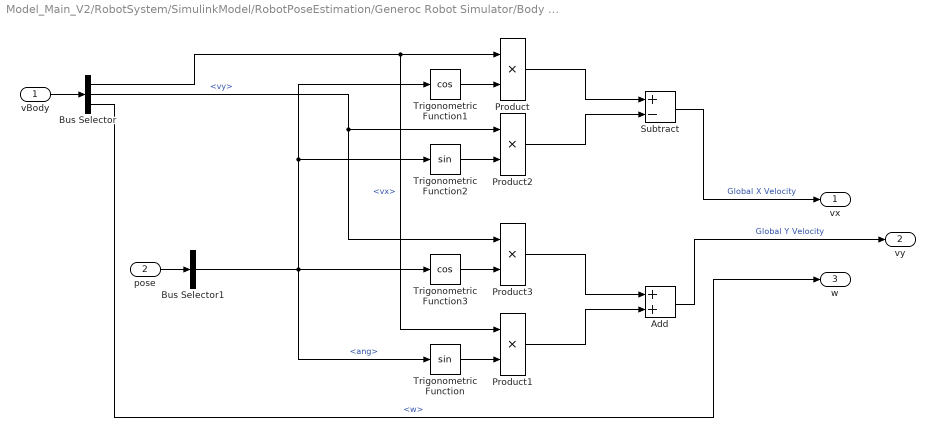
== system Model_Main_V2/RobotSystem/SimulinkModel/RobotPoseEstimation/Generoc Robot Simulator/Body to Cartesian Velocity ==
  vBody : Inport
  pose : Inport  Port=2
  Add : Sum
  Bus Selector : BusSelector  OutputSignals=vx,vy,w
  Bus Selector1 : BusSelector  OutputSignals=ang
  Product{,1..3} (4 alike) : Product
  Subtract : Sum  Inputs=+-
  Trigonometric Function : Trigonometry
  Trigonometric Function1 : Trigonometry  Operator=cos
  Trigonometric Function2 : Trigonometry
  Trigonometric Function3 : Trigonometry  Operator=cos
  vx : Outport  VectorParamsAs1DForOutWhenUnconnected=off
  vy : Outport  Port=2  VectorParamsAs1DForOutWhenUnconnected=off
  w : Outport  Port=3  VectorParamsAs1DForOutWhenUnconnected=off
  wires:
  Bus Selector/3 -> w/1  "<w>"
  vBody/1 -> Bus Selector/1
  Trigonometric Function/1 -> Product1/2
  Product1/1 -> Add/2
  Product/1 -> Subtract/1
  Trigonometric Function1/1 -> Product/2
  Bus Selector/1 -> Product1/1, Product/1  "<vx>"
  Bus Selector1/1 -> Trigonometric Function3/1, Trigonometric Function2/1, Trigonometric Function1/1, Trigonometric Function/1  "<ang>"
  Subtract/1 -> vx/1  "Global X Velocity"
  Trigonometric Function2/1 -> Product2/2
  Bus Selector/2 -> Product3/1, Product2/1  "<vy>"
  Product2/1 -> Subtract/2
  Trigonometric Function3/1 -> Product3/2
  Product3/1 -> Add/1
  Add/1 -> vy/1  "Global Y Velocity"
  pose/1 -> Bus Selector1/1

== system Model_Main_V2/RobotSystem/SimulinkModel/ColorSensor/RegionTracker/LineSubsystem/LineEstimating1 ==
  X : Inport
  Add : Sum
  Constant : Constant  Value=k
  Constant1 : Constant  Value=b
  Product : Product
  Saturation : Saturate  UpperLimit=32  LowerLimit=3
  Color : Outport
  wires:
  Constant1/1 -> Add/2
  Constant/1 -> Product/2
  Add/1 -> Saturation/1
  Product/1 -> Add/1
  X/1 -> Product/1
  Saturation/1 -> Color/1

== matlab function Model_Main_V2/RobotSystem/SimulinkModel/ColorSensor/RegionTracker/RegionTracker/MATLAB Function ==
  data: dot_x input; stateC output; dot_y input
function stateC    =  fcn(dot_x,dot_y)
%create matrix for our point
%Unit of measurement - cm
%properties of lines
%convert meters to cm
dot_x = 100*dot_x ;
dot_y = 100*dot_y;
offset_R = 92.25;
offset_L = 32.25;
line_height_top =59.75;
line_height_bottom = 2.75;
line_width_left = 32.25;
line_width_right = 92.25;
%properties of left circle
CL_height_top = 59.75;
CL_height_bottom = 2.75;
CL_width_left = 0;
CL_width_right = 32.25;
%properties of right circle
CR_height_top = 59.75;
CR_height_bottom = 2.75;
CR_width_left = 92.25;
CR_width_right = 118.8 ;
%Radius
R = 30;
%Estimation of Parameters
p1 = power(dot_x - offset_R,2) + power(dot_y - 30,2); %right circle
p2 = power(dot_x + offset_L - 60,2) + power(dot_y - 30, 2); %left circle
%STATES
%Two lines
state1 = ((line_width_left<dot_x && dot_x<line_width_right) ...
    && ((line_height_bottom<dot_y && dot_y<line_height_top)));
%Right circle
state2 = (((CR_width_left<dot_x && dot_x<CR_width_right) && ...
    ((CR_height_bottom<dot_y && dot_y<CR_height_top)))&&(0<p1 && p1<R^2));
%Left circle
state3 = (((CL_width_left<dot_x && dot_x<CL_width_right) && ...
    ((CL_height_bottom<dot_y && dot_y<CL_height_top)))&&(0<p2 && p2<R^2));

state = state1 | state2 | state3;
if state
    stateC = 32;
else
    stateC = 3;
end

end

== matlab function Model_Main_V2/MATLAB Function2 ==
  data: dot_x input; state output; dot_y input
function state    =  fcn(dot_x,dot_y)
%create matrix for out point
dot = ones(1,2);
dot(1,1) = dot_x(1,1);
dot(1,2) = dot_y(1,1);

%Two lines
X1 = ((-30:30))';
Y1 = 30.*ones(61,1);
Y2 = -Y1;
%check it(two lines)

%right circcle
th = linspace( pi/2, -pi/2, 100);
R = 30;  %or whatever radius you want
x = R*cos(th) + 30;
y = R*sin(th);
%left circle
th2 = linspace( pi/2, 3*pi/2, 100);
R = 30;  %or whatever radius you want
x2 = R*cos(th2) - 30;
y2 = R*sin(th2);
%plotting
p1 = power(dot_x - 0.3,2) + power(dot_y,2);
p2 = power(dot_x + 0.3,2) + power(dot_y,2); 
if (((0.3475<dot_x && dot_x)<0.9495) && ((0.1362<dot_y && dot_y<0.5)) ...%two lines
        ||(((0.0595<dot_x && dot_x<0.3475) && ((0.1362<dot_y && dot_y<0.5)))&&(0<p1 && p1<30)) ...%left circle
        ||(((0.9555<dot_x && dot_x<1.194) && ((0.1362<dot_y && dot_y<0.5)))&&(0<p2 && p2<30))); %right circle
    state = 1;
else
    state = 0;
end
end



% state = (((-30<dot_x && dot_x)<30) && ((-30<dot_y && dot_y<30)) ...%two lines
%         ||(((30<dot_x && dot_x<60) && ((-30<dot_y && dot_y<30)))&&(0<p1 && p1<30)) ...%right circle
%         ||(((-60<dot_x && dot_x<-30) && ((-30<dot_y && dot_y<30)))&&(0<p2 && p2<30))); %left circle
